simulink model "bpsk_rect"  (Simulink 6.4)
settings: Solver=FixedStepDiscrete  StartTime=0.0  StopTime=5  RelTol=1e-3
undefined symbols (not defined in the file or in its folder): Fs, get
libraries: commsink2 x3, commdigbbndpm3 x2, commfilt2 x2, commchan3 x1, dspsrcs4 x1, commrandsrc2 x1, dspsigops x1, dspsnks4 x1
settings Model: Creator=ALEX  LastModifiedBy=student
settings OptimizationCC: InitFltsAndDblsToZero=off
settings DebuggingCC: SignalResolutionControl=UseLocalSettings  MultiTaskDSMMsg=error  MultiTaskCondExecSysMsg=error
settings GRTTargetCC: TargetFcnLib=ansi_tfl_table_tmw.mat

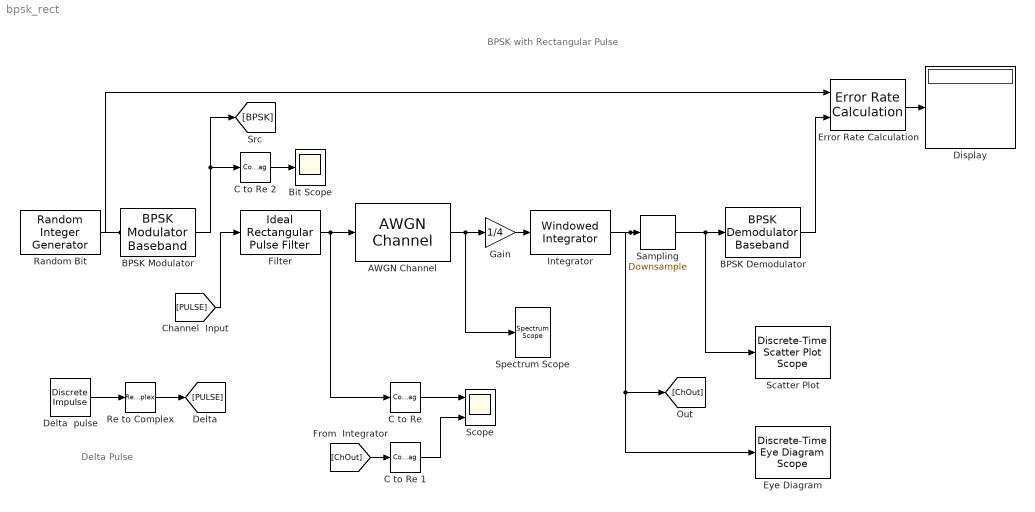
== system bpsk_rect ==
  note: BPSK with Rectangular Pulse
  note: Delta Pulse
  AWGN Channel : commchan3/AWGN Channel  SystemSampleTime=-1  seed=67  noiseMode="Signal to noise ratio  (Es/No)"  EbNodB=3  EsNodB=100  SNRdB=10  bitsPerSym=1  Ps=1/16  Tsym=1  variance=0
  BPSK Demodulator : commdigbbndpm3/BPSK Demodulator Baseband  SystemSampleTime=-1  Ph=0  outDtype=boolean
  BPSK Modulator : commdigbbndpm3/BPSK Modulator Baseband  SystemSampleTime=-1  Ph=0  outDtype=double  outWordLen=16  outUDDataType=sfix(16)  outFracLenMode=Best precision  outFracLen=15
  Bit Scope : Scope
      settings: TimeRange=16  YMin=-1.2  YMax=1.2  SampleTime=1/64
  C to Re : ComplexToRealImag  Output=Real
  C to Re 1 : ComplexToRealImag  Output=Real
  C to Re 2 : ComplexToRealImag  Output=Real
  Delta  pulse : dspsrcs4/Discrete  Impulse  Delay=0  SampleTime=1  FrameSample=1  dataType=double  isSigned=on  wordLen=16  udDataType=sfix(16)  fracBitsMode=Best precision  numFracBits=15
  Display : Display
  Error Rate Calculation : commsink2/Error Rate Calculation  N=2  st_delay=0  cp_mode=Entire frame  subframe=[]  PMode=Port  WsName=ErrorVec  RsMode2=off  stop=off  numErr=100  maxBits=100000
  Eye Diagram : commsink2/Discrete-Time Eye Diagram Scope  Tag=EyeDiagram  SystemSampleTime=-1  sampPerSymb=16  offsetEye=1  symbPerTrace=2  numTraces=50  numNewFrames=5  LineStyles=-  LineColors=r  dupPoints=off  fading=on  render=on  AxisGrid=on  yMin=-2  yMax=2  inphaseLabel=In-phase Amplitude  quadratureLabel=Quadrature Amplitude  openScopeAtSimStart=off  dispDiagram=In-phase Only  FrameNumber=off  FigPos=get(0,'defaultfigureposition');  figTitle=Eye Diagram  block_type_=eye  numLinesMax=8
  Filter : commfilt2/Ideal Rectangular Pulse Filter  SystemSampleTime=-1  pulseLen=16  pulseDelay=0  sampMode=Sample-based  normCheck=on  normMode=Energy per pulse  filterGain=1
  Gain : Gain  Gain=1/4  ParameterDataType=fixdt(1, 16)  OutDataType=fixdt(1, 16)
  Integrator : commfilt2/Windowed Integrator  SystemSampleTime=-1  integperiod=16
  Random Bit : commrandsrc2/Random Integer Generator  SystemSampleTime=-1  mul=2  seed=37  Ts=1  frameBased=off  sampPerFrame=8  orient=off  outDataType=boolean
  "Re to Complex " : RealImagToComplex  Input=Real
  Sampling : dspsigops/Downsample  N=16  phase=15  ic=0  smode=Allow multirate  fmode=Maintain input frame size
  Scatter Plot : commsink2/Discrete-Time Scatter Plot Scope  Tag=ScatterPlot  SystemSampleTime=-1  sampPerSymb=1  offsetEye=0  numTraces=100  numNewFrames=10  LineMarkers=.  LineColors=b  fading=on  render=on  AxisGrid=on  xMin=-2  xMax=2  yMin=-2  yMax=2  inphaseLabel=In-phase Amplitude  quadratureLabel=Quadrature Amplitude  openScopeAtSimStart=off  FrameNumber=off  FigPos=get(0,'defaultfigureposition');  figTitle=Scatter Plot  numLinesMax=8  block_type_=scatter
  Scope : Scope  NumInputPorts=2
      settings: YMin=-0.3~-1.5  YMax=0.3~1.5
  Spectrum Scope : dspsnks4/Spectrum Scope  DialogController=dspdialog.SpectrumScope  DialogControllerArgs=DataTag0  SystemSampleTime=-1  ScopeProperties=on  Domain=Frequency  HorizSpan=1  UseBuffer=on  BufferSize=2048  Overlap=0  inpFftLenInherit=off  FFTlength=128  numAvg=40  DisplayProperties=off  AxisGrid=on  Memory=off  FrameNumber=on  AxisLegend=off  AxisZoom=off  OpenScopeAtSimStart=off  OpenScopeImmediately=off  FigPos=get(0,'defaultfigureposition')  AxisProperties=off  XUnits=Hertz  XRange=[-Fs/2...Fs/2]  InheritXIncr=on  XIncr=1.0  XLabel=Samples  YUnits=dB  YLabel=Magnitude-squared, dB  LineProperties=off  LineStyles=-  LineMarkers=None  LineColors=[1 0 1]  wintypeSpecScope=Hamming  RsSpecScope=50  betaSpecScope=5  winsampSpecScope=Periodic
      settings: YMin=-14.1806  YMax=1.8065
  wires:
  BPSK Demodulator/1 -> Error Rate Calculation/2
  Error Rate Calculation/1 -> Display/1
  C to Re/1 -> Scope/1
  Random Bit/1 -> BPSK Modulator/1, Error Rate Calculation/1
  Filter/1 -> AWGN Channel/1, C to Re/1
  Sampling/1 -> BPSK Demodulator/1, Scatter Plot/1
  Integrator/1 -> Sampling/1, Eye Diagram/1, [ChOut]
  Gain/1 -> Integrator/1
  AWGN Channel/1 -> Gain/1, Spectrum Scope/1
  Delta  pulse/1 -> "Re to Complex "/1
  C to Re 1/1 -> Scope/2
  C to Re 2/1 -> Bit Scope/1
  BPSK Modulator/1 -> C to Re 2/1, [BPSK]
  [PULSE] -> Filter/1
  "Re to Complex "/1 -> [PULSE]
  [ChOut] -> C to Re 1/1
